simulink model "Tez_test_TK"  (R2014a)
settings: Solver=ode4  StartTime=0.0  StopTime=30  FixedStep=0.05  RelTol=1e-3
values from neighbouring files (symbols this model uses):
  K = 1    [RunSim.m]
  Ka = 0.077    [RunSim.m]
  Kb = 7.336    [RunSim.m]
  Kd = 0.5141    [RunSim.m]
  Ke = 1    [RunSim.m]
  L = 0.2    [RunSim.m]
  T = 1    [RunSim.m]
undefined symbols (not defined in the file or in its folder): evalt2
settings Model: Creator=u11f99  LastModifiedBy=Tufan Kumbasar
settings OptimizationCC: ExpressionDepthLimit=2147483647
settings DebuggingCC: UnderspecifiedInitializationDetection=Classic  StateNameClashWarn=warning

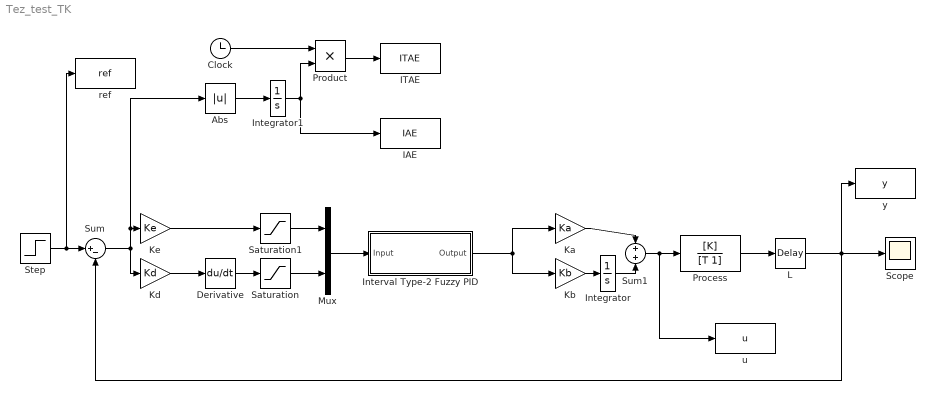
== system Tez_test_TK ==
  Abs : Abs
  Clock : Clock
  Derivative : Derivative
  IAE : ToWorkspace  VariableName=IAE  SaveFormat=Structure With Time  SampleTime=-1
  ITAE : ToWorkspace  VariableName=ITAE  SaveFormat=Structure With Time  SampleTime=-1
  Integrator : Integrator
  Integrator1 : Integrator
  Interval Type-2 Fuzzy PID : Subsystem  AncestorBlock=Fuzzy_Type2_Lib/Interval Type-2 Fuzzy Logic Controller with TR selection  mask(Type-2 Fuzzy Logic Controller){t2fisSim=t2fisSim, TRtype=8}
      mask prompts: t2fisSim "t2fis name in Workspace or File Name"; TRtype "Select TR method"
      mask help:
      | TR Method List for selection;
      |
      | 1 - KM
      | 2 - EKM
      | 3 - IASC
      | 4 - Enhanced Iterative Algorithm With Stop Condition (EIASC)
      | 5 - EODS
      | 6 - WM
      | 7 - NT
      | 8 - BMM
      | 9 - Custom
      mask Display: image(imread('MemberShipMask.jpg'))
  Ka : Gain  Gain=Ka
  Kb : Gain  Gain=Kb
  Kd : Gain  Gain=Kd
  Ke : Gain  Gain=Ke
  L : TransportDelay  DelayTime=L
  Mux : Mux  Inputs=2
  Process : TransferFcn  Numerator=[K]  Denominator=[T 1]
  Product : Product  RndMeth=Zero
  Saturation : Saturate  UpperLimit=1  LowerLimit=-1
  Saturation1 : Saturate  UpperLimit=1  LowerLimit=-1
  Scope : Scope
  Step : Step  SampleTime=0
  Sum : Sum  Inputs=|+-
  Sum1 : Sum
  ref : ToWorkspace  VariableName=ref  SaveFormat=Structure With Time  SampleTime=-1
  u : ToWorkspace  VariableName=u  SaveFormat=Structure With Time  SampleTime=-1
  y : ToWorkspace  VariableName=y  SaveFormat=Structure With Time  SampleTime=-1
  wires:
  Saturation1/1 -> Mux/1
  Saturation/1 -> Mux/2
  Mux/1 -> Interval Type-2 Fuzzy PID/1(Input)
  Derivative/1 -> Saturation/1
  Kd/1 -> Derivative/1
  Ke/1 -> Saturation1/1
  Step/1 -> ref/1, Sum/1
  Sum/1 -> Abs/1, Ke/1, Kd/1
  Interval Type-2 Fuzzy PID/1(Output) -> Kb/1, Ka/1
  Kb/1 -> Integrator/1
  Integrator/1 -> Sum1/2
  Ka/1 -> Sum1/1
  Sum1/1 -> u/1, Process/1
  Process/1 -> L/1
  Abs/1 -> Integrator1/1
  Clock/1 -> Product/1
  Integrator1/1 -> IAE/1, Product/2
  Product/1 -> ITAE/1
  L/1 -> Sum/2, y/1, Scope/1

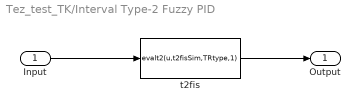
== system Tez_test_TK/Interval Type-2 Fuzzy PID ==
  Input : Inport
  t2fis : MATLABFcn  MATLABFcn=evalt2(u,t2fisSim,TRtype,1)  OutputDimensions=1
  Output : Outport
  wires:
  Input/1 -> t2fis/1
  t2fis/1 -> Output/1
